simulink model "Single_Area"  (Simulink 5.0)
settings: Solver=ode45  StartTime=0.0  StopTime=10.0  RelTol=1e-3
settings Model: LastModifiedBy=MConlon  OptimizeBlockIOStorage=off

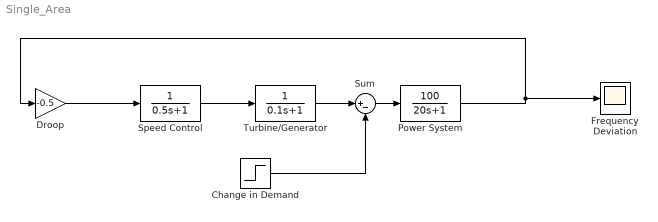
== system Single_Area ==
  Change in Demand : Step  Time=0.0  After=-0.05  SampleTime=0
  Droop : Gain  Gain=-0.5  SaturateOnIntegerOverflow=on
  Frequency Deviation : Scope
  Power System : TransferFcn  Numerator=[100]  Denominator=[20 1]
  Speed Control : TransferFcn  Denominator=[0.5 1]
  Sum : Sum  Inputs=|+-  SaturateOnIntegerOverflow=on
  Turbine/Generator : TransferFcn  Denominator=[0.1 1]
  wires:
  Change in Demand/1 -> Sum/2
  Sum/1 -> Power System/1
  Power System/1 -> Droop/1, Frequency Deviation/1
  Speed Control/1 -> Turbine/Generator/1
  Turbine/Generator/1 -> Sum/1
  Droop/1 -> Speed Control/1
